simulink model "model_test"  (R2024b)
settings: Solver=VariableStepAuto  StartTime=0.0  StopTime=10.0  RelTol=1e-3
settings Model: Creator=mehmetcanevi  LastModifiedBy=mehmetcanevi

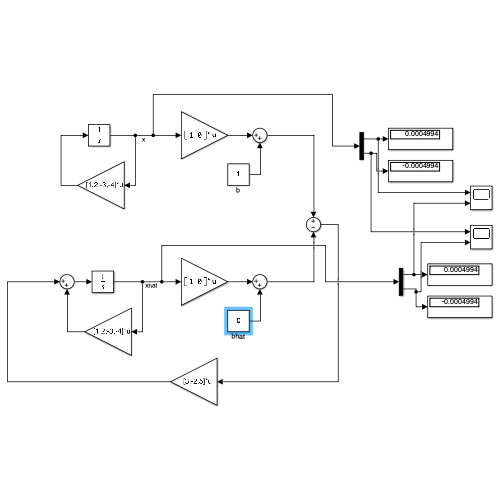
[thumbnail: Simulink's stored preview of the top-level diagram]
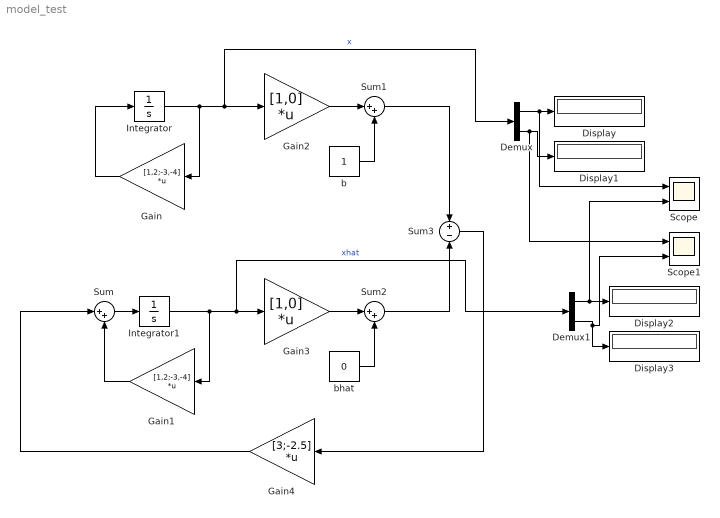
== system model_test ==
  Demux : Demux  Outputs=2
  Demux1 : Demux  Outputs=2
  Display{,1..3} (4 alike) : Display
  Gain : Gain  Gain=[1,2;-3,-4]  Multiplication=Matrix(K*u)
  Gain1 : Gain  Gain=[1,2;-3,-4]  Multiplication=Matrix(K*u)
  Gain2 : Gain  Gain=[1,0]  Multiplication=Matrix(K*u)
  Gain3 : Gain  Gain=[1,0]  Multiplication=Matrix(K*u)
  Gain4 : Gain  Gain=[3;-2.5]  Multiplication=Matrix(K*u)
  Integrator : Integrator  InitialCondition=[3;1]
  Integrator1 : Integrator
  Scope : Scope  NumInputPorts=2
  Scope1 : Scope  NumInputPorts=2
  Sum : Sum  Inputs=|++
  Sum1 : Sum  Inputs=|++
  Sum2 : Sum  Inputs=|++
  Sum3 : Sum  Inputs=+-
  b : Constant
  bhat : Constant  Value=0
  wires:
  Gain/1 -> Integrator/1
  Integrator/1 -> Demux/1, Gain2/1, Gain/1  "x"
  Sum/1 -> Integrator1/1
  Gain1/1 -> Sum/2
  Gain2/1 -> Sum1/1
  b/1 -> Sum1/2
  bhat/1 -> Sum2/2
  Gain3/1 -> Sum2/1
  Sum1/1 -> Sum3/1
  Sum2/1 -> Sum3/2
  Sum3/1 -> Gain4/1
  Gain4/1 -> Sum/1
  Demux/1 -> Scope/1, Display/1
  Demux/2 -> Scope1/1, Display1/1
  Demux1/2 -> Scope1/2, Display3/1
  Integrator1/1 -> Demux1/1, Gain3/1, Gain1/1  "xhat"
  Demux1/1 -> Scope/2, Display2/1
